simulink model "JGVD_Mixing_Tank"  (R2022a)
settings: Solver=VariableStepAuto  StartTime=0.0  StopTime=200  RelTol=1e-3
values from neighbouring files (symbols this model uses):
  seedPI = 3    [JGVD_Mixing_Tank_Parameters.m]    (also in JGVD_Non_Isothermal_CSTR_Parameters.m)
  varPI = 5E-5    (= 5e-05)    [JGVD_Mixing_Tank_Parameters.m]    (also in JGVD_Non_Isothermal_CSTR_Parameters.m)
  xA = ((p.F1 + p.F2)*xA_0)/(p.F1 + p.F2)    [JGVD_Mixing_Tank_Parameters.m]
undefined symbols (not defined in the file or in its folder): p
settings Model: Creator=18279724  LastModifiedBy=georg
settings SolverCC: AlgebraicLoopSolver=TrustRegion
settings DataIOCC: ReturnWorkspaceOutputs=off
settings DebuggingCC: UnconnectedInputMsg=warning  UnconnectedOutputMsg=warning  UnconnectedLineMsg=warning  SFMachineParentedDataDiag=warning  ArithmeticOperatorsInVariantConditions=warning
settings SFSimCC: SimUseLocalCustomCode=off  CustomCodeUndefinedFunction=UseInterfaceOnly
settings RTWCC: RTWUseLocalCustomCode=off

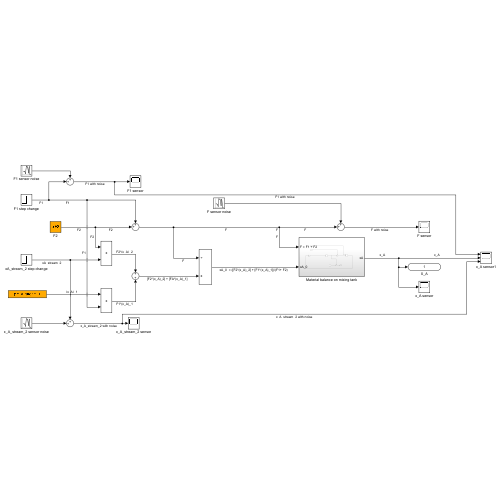
[thumbnail: Simulink's stored preview of the top-level diagram]
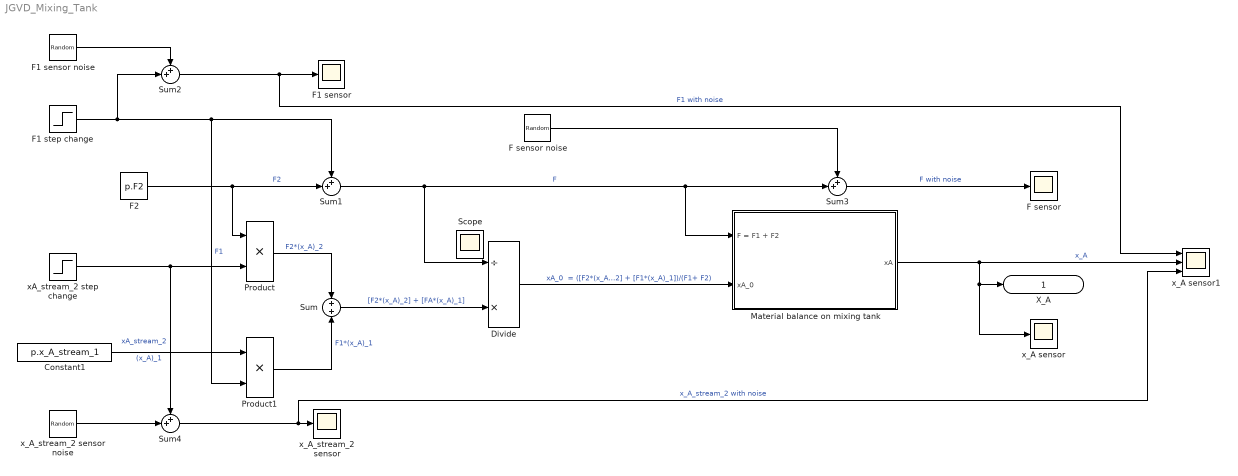
== system JGVD_Mixing_Tank ==
  Constant1 : Constant  Value=p.x_A_stream_1
  Divide : Product  Inputs=/*
  F sensor : Scope
  F sensor noise : RandomNumber  Variance=varPI  Seed=seedPI  SampleTime=0.1
  F1 sensor : Scope
  F1 sensor noise : RandomNumber  Variance=varPI  Seed=seedPI  SampleTime=0.1
  F1 step change : Step  Time=20  Before=p.F1  After=p.F1  SampleTime=0
  F2 : Constant  Value=p.F2
  Material balance on mixing tank : Subsystem
  Product : Product
  Product1 : Product
  Sum : Sum
  Sum{1..4} (4 alike) : Sum  Inputs=++|
  xA_stream_2 step change : Step  Time=20  Before=p.x_A_stream_2  After=p.x_A_stream_2*2  SampleTime=0
  x_A sensor : Scope
  x_A sensor1 : Scope  NumInputPorts=3
  x_A_stream_2 sensor : Scope
  x_A_stream_2 sensor noise : RandomNumber  Variance=varPI  Seed=seedPI  SampleTime=0.1
  X_A : Outport  VectorParamsAs1DForOutWhenUnconnected=off
  Scope : Scope
  wires:
  F2/1 -> Product/1, Sum1/2  "F2"
  xA_stream_2 step change/1 -> Product/2, Sum4/1  "xA_stream_2"
  Constant1/1 -> Product1/1  "(x_A)_1"
  Material balance on mixing tank/1(xA) -> x_A sensor1/2, x_A sensor/1, X_A/1  "x_A"
  Sum1/1 -> Material balance on mixing tank/1(F = F1 + F2), Sum3/2, Divide/1  "F"
  F1 step change/1 -> Product1/2, Sum1/1, Sum2/2  "F1"
  F1 sensor noise/1 -> Sum2/1
  Sum2/1 -> x_A sensor1/1, F1 sensor/1  "F1 with noise"
  F sensor noise/1 -> Sum3/1
  Sum3/1 -> F sensor/1  "F with noise"
  x_A_stream_2 sensor noise/1 -> Sum4/2
  Sum4/1 -> x_A sensor1/3, x_A_stream_2 sensor/1  "x_A_stream_2 with noise"
  Divide/1 -> Material balance on mixing tank/2("xA_0 ")  "xA_0  = ([F2*(x_A)_2] + [F1*(x_A)_1])/(F1+ F2)"
  Product1/1 -> Sum/2  "F1*(x_A)_1"
  Sum/1 -> Divide/2  "[F2*(x_A)_2] + [FA*(x_A)_1]"
  Product/1 -> Sum/1  "F2*(x_A)_2"

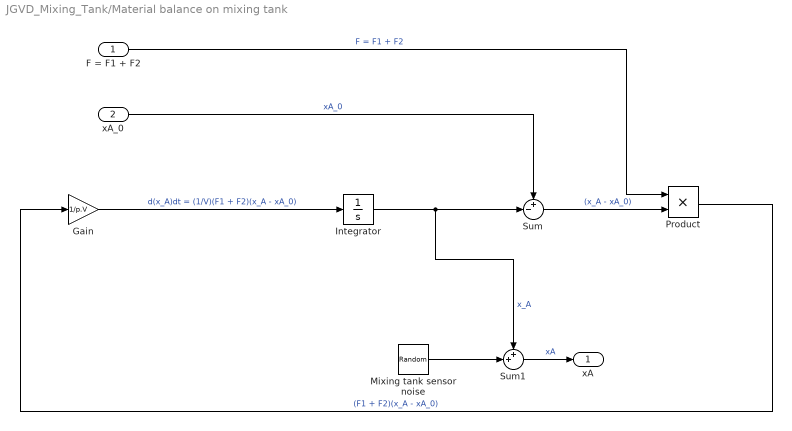
== system JGVD_Mixing_Tank/Material balance on mixing tank ==
  F = F1 + F2 : Inport
  "xA_0 " : Inport  Port=2
  Gain : Gain  Gain=1/p.V
  Integrator : Integrator  InitialCondition=xA
  Mixing tank sensor noise : RandomNumber  Variance=varPI  Seed=seedPI  SampleTime=0.1
  Product : Product
  Sum : Sum  Inputs=+-|
  Sum1 : Sum  Inputs=++|
  xA : Outport  VectorParamsAs1DForOutWhenUnconnected=off
  wires:
  Sum1/1 -> xA/1  "xA"
  Mixing tank sensor noise/1 -> Sum1/2
  "xA_0 "/1 -> Sum/1  "xA_0"
  Sum/1 -> Product/2  "(x_A - xA_0)"
  F = F1 + F2/1 -> Product/1  "F = F1 + F2"
  Product/1 -> Gain/1  "(F1 + F2)(x_A - xA_0)"
  Integrator/1 -> Sum/2, Sum1/1  "x_A"
  Gain/1 -> Integrator/1  "d(x_A)dt = (1/V)(F1 + F2)(x_A - xA_0)"
